simulink model "Q1"  (R2018a)
settings: Solver=FixedStepAuto  StartTime=0.0  StopTime=10  RelTol=1e-3
libraries: powerlib x13, powerlib_meascontrol x2, halfcontrolled x1
settings Model: Creator=nailt  LastModifiedBy=nailt

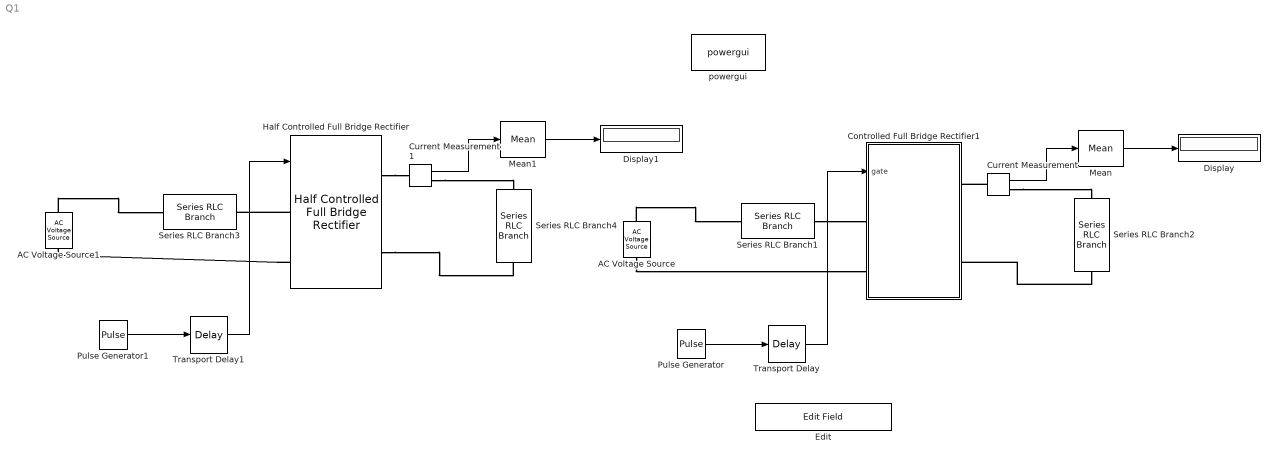
== system Q1 ==
  AC Voltage Source : powerlib/Electrical Sources/AC Voltage Source  Amplitude=230*sqrt(2)  Phase=0  Frequency=50  SampleTime=0  Measurements=None  BusType=swing  Pref=10e3  Qref=0  Qmin=-inf  Qmax=+inf
  AC Voltage Source1 : powerlib/Electrical Sources/AC Voltage Source  Amplitude=230*sqrt(2)  Phase=0  Frequency=50  SampleTime=0  Measurements=None  BusType=swing  Pref=10e3  Qref=0  Qmin=-inf  Qmax=+inf
  Controlled Full Bridge Rectifier1 : Subsystem  AncestorBlock=halfcontrolled/Controlled Full Bridge Rectifier
  Current Measurement : powerlib/Measurements/Current Measurement  PhasorSimulation=off  OutputType=Complex  PSBequivalent=0
  Current Measurement1 : powerlib/Measurements/Current Measurement  PhasorSimulation=off  OutputType=Complex  PSBequivalent=0
  Display : Display
  Display1 : Display
  Edit : EditField  WebBlockId=182  LabelPosition=Hide  Alignment=Center
  Half Controlled Full Bridge Rectifier : halfcontrolled/Half Controlled Full Bridge Rectifier
  Mean : powerlib_meascontrol/Measurements/Mean  Freq=50  Vinit=0  Ts=0
  Mean1 : powerlib_meascontrol/Measurements/Mean  Freq=50  Vinit=0  Ts=0
  Pulse Generator : DiscretePulseGenerator  PulseType=Time based  Period=0.02  PulseWidth=10
  Pulse Generator1 : DiscretePulseGenerator  PulseType=Time based  Period=0.02  PulseWidth=10
  Series RLC Branch1 : powerlib/Elements/Series RLC Branch  LConnTagsString=__new0  RConnTagsString=__new0  BranchType=L  Resistance=4  Inductance=0.5e-3  SetiL0=off  InitialCurrent=0  Capacitance=1e-6  Setx0=off  InitialVoltage=0  Measurements=None
  Series RLC Branch2 : powerlib/Elements/Series RLC Branch  LConnTagsString=__new0  RConnTagsString=__new0  BranchType=RL  Resistance=4  Inductance=200e-6  SetiL0=off  InitialCurrent=0  Capacitance=1e-6  Setx0=off  InitialVoltage=0  Measurements=None
  Series RLC Branch3 : powerlib/Elements/Series RLC Branch  LConnTagsString=__new0  RConnTagsString=__new0  BranchType=L  Resistance=4  Inductance=0.5e-3  SetiL0=off  InitialCurrent=0  Capacitance=1e-6  Setx0=off  InitialVoltage=0  Measurements=None
  Series RLC Branch4 : powerlib/Elements/Series RLC Branch  LConnTagsString=__new0  RConnTagsString=__new0  BranchType=RL  Resistance=4  Inductance=200e-6  SetiL0=off  InitialCurrent=0  Capacitance=1e-6  Setx0=off  InitialVoltage=0  Measurements=None
  Transport Delay : TransportDelay  DelayTime=0.02*37.53/360
  Transport Delay1 : TransportDelay  DelayTime=0.02*55/360
  powergui : powerlib/powergui  Priority=1  SimulationMode=Discrete  SampleTime=50e-7  frequency=60  Iterations=50  frequencyindice=0  Pbase=100e6  ErrMax=1e-4  UnitsV=kV  UnitsW=MW  buscounter=0  FunctionMessages=off  echomessages=off  EnableUseOfTLC=off  CurrentSourceSwitches=off  DisableSnubberDevices=off  DisableRonSwitches=off  DisableVfSwitches=off  DisplayEquations=off  SolverType=Tustin/Backward Euler (TBE)  Interpol=off  ExternalGateDelay=off  methode=off  Ts=100  x0status=blocks  SPID=off  SwTol=0  HookPort=off  RestoreLinks=warning  ResistiveCurrentMeasurement=off  Frange=[0:2:500]  Ylog=off  Xlog=on  ShowGrid=off  save=off  variable=ZData  structure=simout  ZoomFFT=off  StartTime=0.0  cycles=3  DisplayStyle=1  fundamental=50  FreqAxis=off  MaxFrequency=1000  frequencyindicesteady=1  RmsSteady=1  display=off
  wires:
  Pulse Generator/1 -> Transport Delay/1
  Transport Delay/1 -> Controlled Full Bridge Rectifier1/1(gate)
  Current Measurement/1 -> Mean/1
  Mean/1 -> Display/1
  Current Measurement1/1 -> Mean1/1
  Mean1/1 -> Display1/1
  Transport Delay1/1 -> Half Controlled Full Bridge Rectifier/1
  Pulse Generator1/1 -> Transport Delay1/1
  connections:
  AC Voltage Source/LConn1 -- Controlled Full Bridge Rectifier1/LConn2
  Series RLC Branch1/RConn1 -- Controlled Full Bridge Rectifier1/LConn1
  Series RLC Branch2/RConn1 -- Controlled Full Bridge Rectifier1/RConn2
  AC Voltage Source/RConn1 -- Series RLC Branch1/LConn1
  Current Measurement/LConn1 -- Controlled Full Bridge Rectifier1/RConn1
  Current Measurement/RConn1 -- Series RLC Branch2/LConn1
  Half Controlled Full Bridge Rectifier/RConn2 -- Series RLC Branch4/RConn1
  Current Measurement1/RConn1 -- Series RLC Branch4/LConn1
  Half Controlled Full Bridge Rectifier/LConn2 -- AC Voltage Source1/LConn1
  Half Controlled Full Bridge Rectifier/RConn1 -- Current Measurement1/LConn1
  Half Controlled Full Bridge Rectifier/LConn1 -- Series RLC Branch3/RConn1
  AC Voltage Source1/RConn1 -- Series RLC Branch3/LConn1

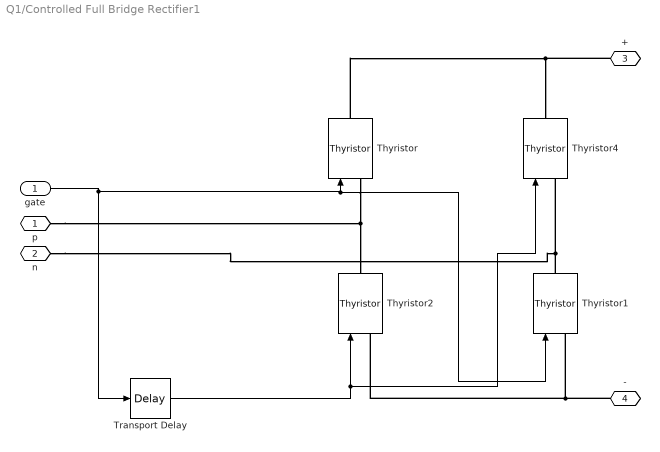
== system Q1/Controlled Full Bridge Rectifier1 ==
  gate : Inport
  Thyristor{,1..2,4} (4 alike) : powerlib/Power Electronics/Thyristor  Ron=0.00001  Lon=0  Vf=0  IC=0  Rs=10e9  Cs=250e-12  Measurements=off
  Transport Delay : TransportDelay  DelayTime=0.01
  p : PMIOPort  Side=Left
  n : PMIOPort  Port=2  Side=Left
  + : PMIOPort  Port=3  Side=Right
  - : PMIOPort  Port=4  Side=Right
  wires:
  gate/1 -> Thyristor1/1, Thyristor/1, Transport Delay/1
  Transport Delay/1 -> Thyristor4/1, Thyristor2/1
  connections:
  -/RConn1 -- Thyristor2/LConn1 -- Thyristor1/LConn1
  Thyristor1/RConn1 -- n/RConn1 -- Thyristor4/LConn1
  Thyristor/LConn1 -- p/RConn1 -- Thyristor2/RConn1
  +/RConn1 -- Thyristor/RConn1 -- Thyristor4/RConn1
